simulink model "renewable_energy_assignment1_part4"  (R2026a)
settings: Solver=VariableStepAuto  StopTime=100
settings Model: Creator=zeyneptutumlu

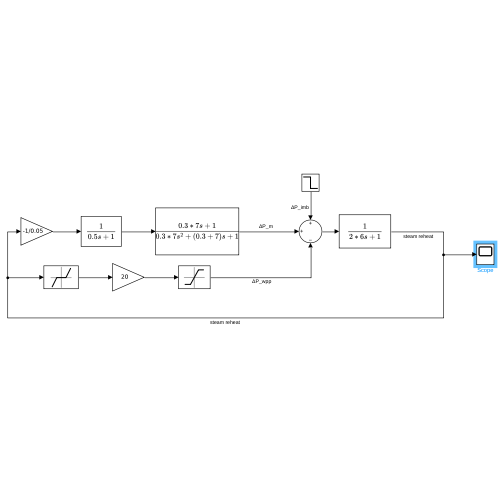
[thumbnail: Simulink's stored preview of the top-level diagram]
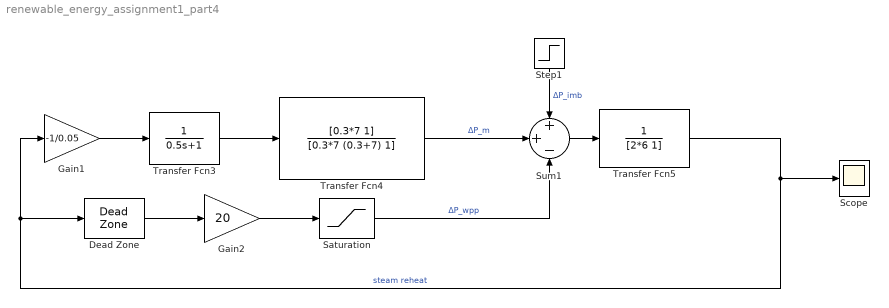
== system renewable_energy_assignment1_part4 ==
  Dead Zone : DeadZone  LowerValue=-0.001  UpperValue=0.001
  Gain1 : Gain  Gain=-1/0.05
  Gain2 : Gain  Gain=20
  Saturation : Saturate  UpperLimit=0.2  LowerLimit=-0.2
  Scope : Scope
      settings: ActiveDisplayYMinimum=-0.01410788861959272  ActiveDisplayYMaximum=0.0048342168745356849
  Step1 : Step  FinalValue=-0.1  SampleTime=0
  Sum1 : Sum  Inputs=++-
  Transfer Fcn3 : TransferFcn  Denominator=[0.5 1]
  Transfer Fcn4 : TransferFcn  Numerator=[0.3*7 1]  Denominator=[0.3*7 (0.3+7) 1]
  Transfer Fcn5 : TransferFcn  Denominator=[2*6 1]
  wires:
  Step1/1 -> Sum1/1  "ΔP_imb"
  Transfer Fcn5/1 -> Dead Zone/1, Gain1/1, Scope/1  "steam reheat"
  Gain1/1 -> Transfer Fcn3/1
  Transfer Fcn4/1 -> Sum1/2  "ΔP_m"
  Sum1/1 -> Transfer Fcn5/1
  Transfer Fcn3/1 -> Transfer Fcn4/1
  Dead Zone/1 -> Gain2/1
  Gain2/1 -> Saturation/1
  Saturation/1 -> Sum1/3  "ΔP_wpp"
